simulink model "AnalogChannel"  (R2023a)
settings: Solver=VariableStepAuto  StartTime=0.0  StopTime=10  RelTol=1e-3
libraries: dspfdesign x3, dspmathops x2, dspsrcs4 x1
settings Model: Creator=PANKAJA  LastModifiedBy=PANKAJA

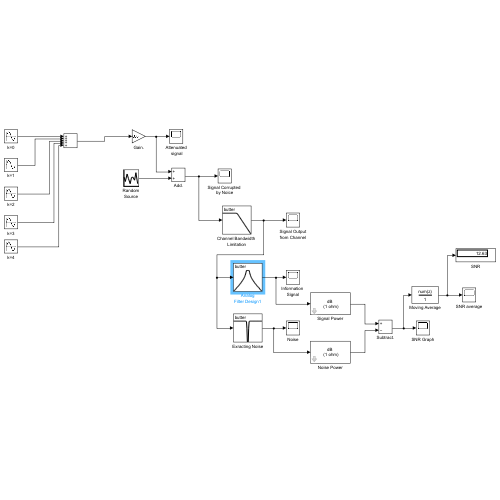
[thumbnail: Simulink's stored preview of the top-level diagram]
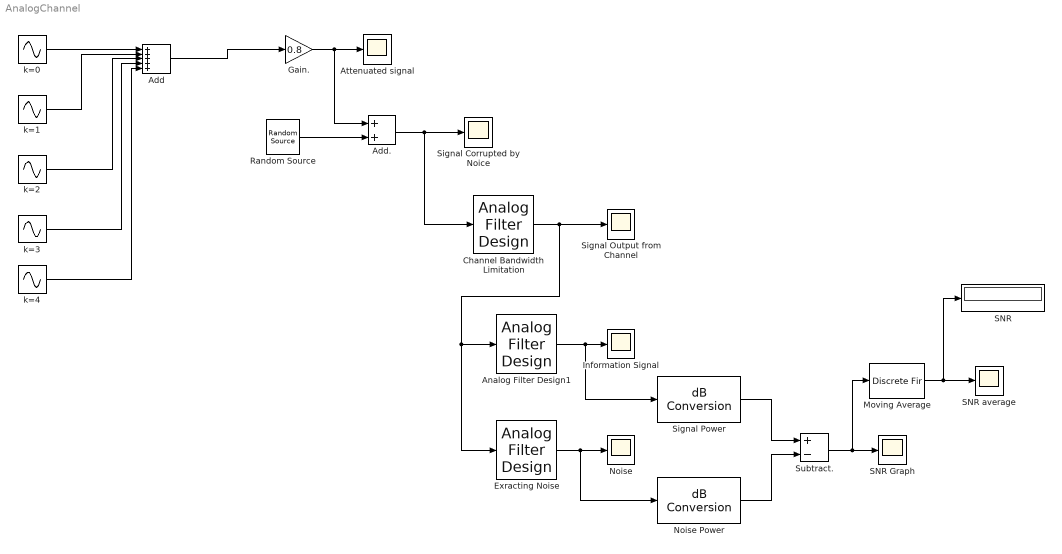
== system AnalogChannel ==
  Add : Sum  Inputs=+++++
  Add. : Sum
  Analog Filter Design1 : dspfdesign/Analog Filter Design  method=Butterworth  filttype=Bandpass  N=10  Wlo=195  Whi=285  Rp=2  Rs=40
  Attenuated signal : Scope
  Channel Bandwidth Limitation : dspfdesign/Analog Filter Design  method=Butterworth  filttype=Lowpass  N=10  Wlo=1000  Whi=80  Rp=2  Rs=40
  Exracting Noise : dspfdesign/Analog Filter Design  method=Butterworth  filttype=Bandstop  N=10  Wlo=195  Whi=285  Rp=2  Rs=40
  Gain. : Gain  Gain=0.8
  Information Signal : Scope
  Moving Average : DiscreteFir  Coefficients=ones(1,1000)/1000  SampleTime=0.001
  Noise : Scope
  Noise Power : dspmathops/dB Conversion  dBtype=dB  intype=Amplitude  R=1  fuzz=off
      settings: LibrarySourceBlock=commutil2/dB Conversion
  Random Source : dspsrcs4/Random Source  SrcType=Gaussian  NormMethod=Ziggurat  CltLength=12  MinVal=0  MaxVal=1  MeanVal=0  VarVal=1  RepMode=Not repeatable  rawSeed=1  IsInherit=off  SampMode=Discrete  SampTime=0.001  SampFrame=1  DataType=Double  OutComplex=Real  OutputFrames=off
  SNR : Display
  SNR Graph : Scope
  SNR average : Scope
  Signal Corrupted by Noice : Scope
  Signal Output from Channel : Scope
  Signal Power : dspmathops/dB Conversion  dBtype=dB  intype=Amplitude  R=1  fuzz=off
      settings: LibrarySourceBlock=commutil2/dB Conversion
  Subtract. : Sum  Inputs=+-
  k=0 : Sin  Amplitude=10  Frequency=200  SampleTime=0
  k=1 : Sin  Amplitude=8  Frequency=220  SampleTime=0
  k=2 : Sin  Amplitude=6  Frequency=240  SampleTime=0
  k=3 : Sin  Amplitude=4  Frequency=260  SampleTime=0
  k=4 : Sin  Amplitude=2  Frequency=280  SampleTime=0
  wires:
  Gain./1 -> Add./1, Attenuated signal/1
  Random Source/1 -> Add./2
  Add./1 -> Channel Bandwidth Limitation/1, Signal Corrupted by Noice/1
  Channel Bandwidth Limitation/1 -> Exracting Noise/1, Analog Filter Design1/1, Signal Output from Channel/1
  Analog Filter Design1/1 -> Signal Power/1, Information Signal/1
  Exracting Noise/1 -> Noise Power/1, Noise/1
  Noise Power/1 -> Subtract./2
  Signal Power/1 -> Subtract./1
  Subtract./1 -> Moving Average/1, SNR Graph/1
  Moving Average/1 -> SNR/1, SNR average/1
  k=0/1 -> Add/1
  k=1/1 -> Add/2
  k=2/1 -> Add/3
  k=3/1 -> Add/4
  k=4/1 -> Add/5
  Add/1 -> Gain./1
